simulink model "multicarFS_spacingError"  (R2019a)
settings: Solver=FixedStepAuto  StartTime=0.0  StopTime=600  FixedStep=0.01  RelTol=1e-3
libraries: simulink x14, autolibshared x8, vehdynlibsteering x8, autolibutils x8, eeGeneralControl x7
(part 1 of 2)
settings Model: Creator=ckreienk  LastModifiedBy=ckreienk

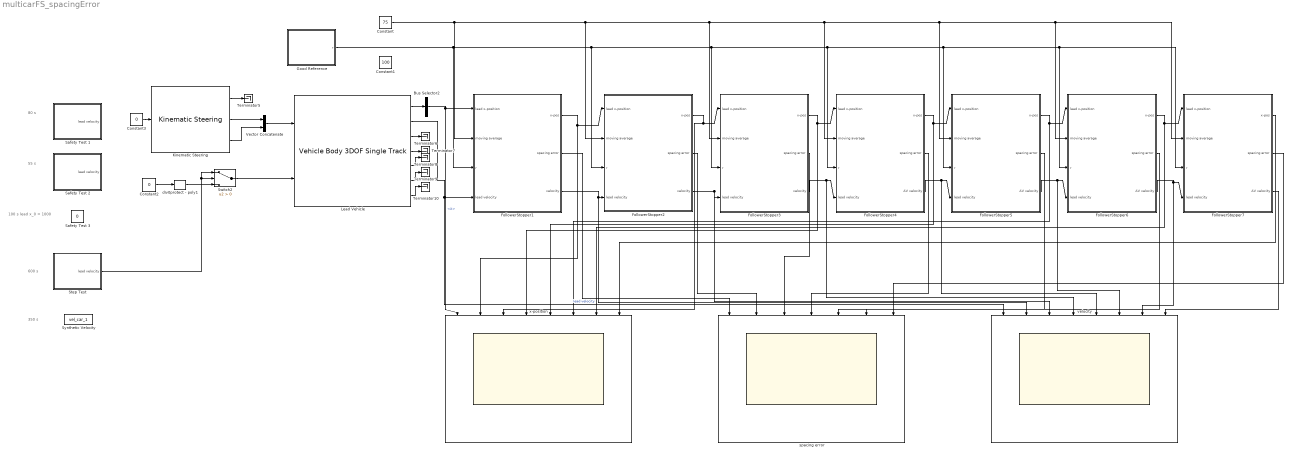
== system multicarFS_spacingError ==
  note: 600 s
  note: 100 s
      | lead x_0 = 1000
  note: 55 s
  note: 350 s
  note: 80 s
  Bus Selector2 : BusSelector  OutputSignals=InertFrm.Geom.Disp.X
  Constant : Constant  Value=75
  Constant1 : Constant  Value=100
  Constant2 : Constant  Value=0
  Constant3 : Constant  Value=0
  FollowerStopper1 : Subsystem
  FollowerStopper2 : Subsystem
  FollowerStopper3 : Subsystem
  FollowerStopper4 : Subsystem
  FollowerStopper5 : Subsystem
  FollowerStopper6 : Subsystem
  FollowerStopper7 : Subsystem
  Good Reference : Subsystem
  Kinematic Steering : vehdynlibsteering/Kinematic Steering  StrgType=Ackerman  StrgRatioType=Constant  Loc=Front  NrmlFctr=0.01  TrckWdth=1  WhlBase=1.524  Db=0  StrgRng=1.25*pi  StrgAngBpts="[-6.2832   -5.0265   -3.7699   -2.5133   -1.2566         0    1.2566    2.5133    3.7699    5.0265    6.2832]"  StrgRatioTbl=|  StrgRatio=100  StrgArmLngth=0.1  RckCsLngth=0.5  TieRodLngth=0.248  D=0.2  PnnRadius=0.0057  PnnRadiusTbl="[0.0055    0.0055    0.0056    0.0057    0.0058    0.0057    0.0057    0.0057    0.0056    0.0055    0.0055]"  RodLngth=0.1  ParaArmLngth=0.9  aMode=2
      | [13.5000   13.3750   13.2500   13.1250   13.0000   13.0000   13.0000   13.1250   13.2500   13.3750   13.5000
      | ]
      settings: SourceProductName=Vehicle Dynamics Blockset
  Lead Vehicle : autolibshared/Vehicle Body 3DOF Single Track  trackMode=Dual  inputMode=External longitudinal velocity  frontSteerMode=on  rearSteerMode=off  windMode=off  muMode=off  extFMode=off  extMMode=off  extXo=off  extpsio=off  extxdoto=off  extro=off  extYo=off  extTamb=off  extydoto=off  aMode=2  NF=2  NR=2  m=2000  a=1.4  b=1.6  h=0.35  X_o=80  xdot_o=0  CalphaMode=off  sigmaMode=on  d=0  w=[1.4,1.4]  Cy_f=12e3  Cy_r=11e3  sigma_f=.1  sigma_r=.1  alpha_f_brk=[-.1 .1]  Cy_f_data=[-9e3 9e3]  alpha_r_brk=[-.1 .1]  Cy_r_data=[-9e3 9e3]  Y_o=0  ydot_o=0  Izz=4000  psi_o=0  r_o=0  Af=2  Cd=.3  Cl=.1  Cpm=.1  beta_w=[0:0.01:0.3]  Cs=[0:0.03:0.9]  Cym=[0:0.01:0.3]  Pabs=101325  Tair=273  g=9.81  mu=1  xdot_tol=.01  Fznom=5000  Fxtire_sat=7e4  Fytire_sat=7e4  longOff=0  latOff=0  vertOff=0  wrapAng=off
      settings: SourceProductName=Powertrain Blockset  SourceProductBaseCode=PW
  Safety Test 1 : Subsystem
  Safety Test 2 : Subsystem
  Safety Test 3 : Constant  Value=0
  Step Test : Subsystem
  Switch2 : Switch  Criteria=u2 > Threshold
  Synthetic Velocity : FromWorkspace  VariableName=vel_car_1
  Terminator{5..10} (6 alike) : Terminator
  Vector Concatenate : Concatenate
  div0protect - poly1 : autolibutils/div0protect - poly  thresh=1e-3  aMode=2
      settings: SourceProductName=Powertrain Blockset  SourceProductBaseCode=PW
  spacing error : Scope  NumInputPorts=7
  velocity : Scope  NumInputPorts=8
  x-position : Scope  NumInputPorts=8
  wires:
  Constant3/1 -> Kinematic Steering/1
  Switch2/1 -> Lead Vehicle/2
  Kinematic Steering/3 -> Vector Concatenate/2
  div0protect - poly1/1 -> Switch2/3
  Lead Vehicle/6 -> Terminator9/1
  Step Test/1(lead velocity) -> Switch2/1, Switch2/2
  Kinematic Steering/2 -> Vector Concatenate/1
  Lead Vehicle/7 -> Terminator10/1
  Lead Vehicle/3 -> Terminator6/1
  Lead Vehicle/4 -> Terminator7/1
  Constant2/1 -> div0protect - poly1/1
  Kinematic Steering/1 -> Terminator5/1
  Vector Concatenate/1 -> Lead Vehicle/1
  Lead Vehicle/2 -> velocity/1, FollowerStopper1/4(lead velocity)  "lead velocity"
  Lead Vehicle/5 -> Terminator8/1
  Bus Selector2/1 -> FollowerStopper1/1(lead x-position), x-position/1  "<X>"
  Lead Vehicle/1 -> Bus Selector2/1
  FollowerStopper1/1(x-pos) -> x-position/2, FollowerStopper2/1(lead x-position)
  FollowerStopper1/3(velocity) -> velocity/2, FollowerStopper2/4(lead velocity)
  FollowerStopper2/1(x-pos) -> x-position/3, FollowerStopper3/1(lead x-position)
  FollowerStopper2/3(velocity) -> FollowerStopper3/4(lead velocity), velocity/3
  FollowerStopper3/1(x-pos) -> x-position/4, FollowerStopper4/1(lead x-position)
  FollowerStopper3/3(velocity) -> velocity/4, FollowerStopper4/4(lead velocity)
  FollowerStopper4/1(x-pos) -> x-position/5, FollowerStopper5/1(lead x-position)
  FollowerStopper4/3(AV velocity) -> velocity/5, FollowerStopper5/4(lead velocity)
  FollowerStopper5/1(x-pos) -> x-position/6, FollowerStopper6/1(lead x-position)
  FollowerStopper5/3(AV velocity) -> velocity/6, FollowerStopper6/4(lead velocity)
  FollowerStopper6/1(x-pos) -> x-position/7, FollowerStopper7/1(lead x-position)
  FollowerStopper6/3(AV velocity) -> velocity/7, FollowerStopper7/4(lead velocity)
  FollowerStopper7/1(x-pos) -> x-position/8
  FollowerStopper6/2(spacing error) -> spacing error/6
  FollowerStopper3/2(spacing error) -> spacing error/3
  FollowerStopper2/2(spacing error) -> spacing error/2
  FollowerStopper5/2(spacing error) -> spacing error/5
  FollowerStopper7/2(spacing error) -> spacing error/7
  FollowerStopper1/2(spacing error) -> spacing error/1
  FollowerStopper4/2(spacing error) -> spacing error/4
  FollowerStopper7/3(AV velocity) -> velocity/8
  Constant/1 -> FollowerStopper7/2(moving average), FollowerStopper6/2(moving average), FollowerStopper5/2(moving average), FollowerStopper4/2(moving average), FollowerStopper3/2(moving average), FollowerStopper2/2(moving average), FollowerStopper1/2(moving average)
  Good Reference/1(r) -> FollowerStopper6/3(r), FollowerStopper7/3(r), FollowerStopper5/3(r), FollowerStopper4/3(r), FollowerStopper3/3(r), FollowerStopper2/3(r), FollowerStopper1/3(r)

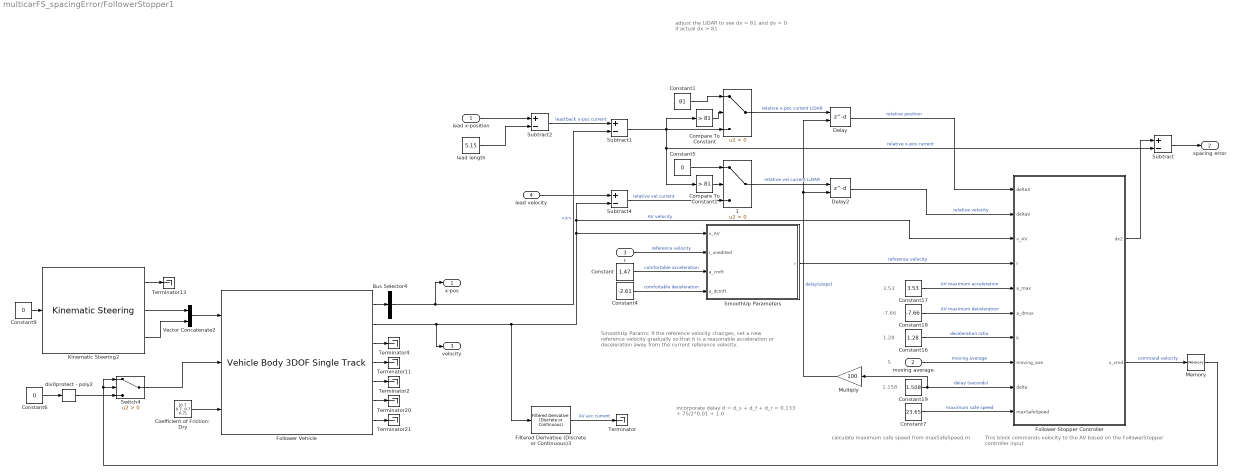
== system multicarFS_spacingError/FollowerStopper1 ==
  note: -7.66
  note: 5
  note: 1.158
  note: adjust the LiDAR to see
      | dx = 81 and dv = 0
      | if actual dx > 81
  note: incorporate delay
      | d = d_s + d_f + d_r
      | = 0.133 + 75/2*0.01 + 1.0
  note: SmoothUp Params:
      | If the reference velocity changes,
      | set a new reference velocity gradually
      | so that it is a reasonable acceleration
      | or deceleration away from the current
      | reference velocity.
  note: This block commands velocity to the AV based
      | on the FollowerStopper controller input
  note: calculate maximum safe speed
      | from maxSafeSpeed.m
  note: 3.53
  note: 1.28
  lead x-position : Inport
  moving average : Inport  Port=2
  r : Inport  Port=3
  lead velocity : Inport  Port=4
  " " : Switch  Criteria=u2 > Threshold
  " 1" : Switch  Criteria=u2 > Threshold
  Bus Selector4 : BusSelector  OutputSignals=InertFrm.Geom.Disp.X
  Coefficient of Friction: Dry : Constant  Value=[0.7 0.7; 0.7 0.7]
  Compare To Constant : simulink/Logic and Bit Operations/Compare To Constant  relop=>  const=81  OutDataTypeStr=boolean
  Compare To Constant1 : simulink/Logic and Bit Operations/Compare To Constant  relop=>  const=81  OutDataTypeStr=boolean
  Constant : Constant  Value=1.47
  Constant1 : Constant  Value=81
  Constant16 : Constant  Value=1.28
  Constant17 : Constant  Value=3.53
  Constant18 : Constant  Value=-7.66
  Constant19 : Constant  Value=1.508
  Constant4 : Constant  Value=-2.61
  Constant5 : Constant  Value=0
  Constant6 : Constant  Value=0
  Constant7 : Constant  Value=23.65
  Constant9 : Constant  Value=0
  Delay : Delay  DelayLengthSource=Input port  DelayLength=183
      settings: InputPortMap=u0,p1
  Delay2 : Delay  DelayLengthSource=Input port  DelayLength=183
      settings: InputPortMap=u0,p1
  Filtered Derivative (Discrete or Continuous)3 : eeGeneralControl/Filtered Derivative (Discrete or Continuous)  K=1  T=0.1  B=20  A=-20  minRatio=10  Ts=-1
      settings: SourceProductName=Simscape Electrical  SourceProductBaseCode=PS
  Follower Stopper Controller : Subsystem
  Follower Vehicle : autolibshared/Vehicle Body 3DOF Single Track  trackMode=Dual  inputMode=External longitudinal velocity  frontSteerMode=on  rearSteerMode=off  windMode=off  muMode=on  extFMode=off  extMMode=off  extXo=off  extpsio=off  extxdoto=off  extro=off  extYo=off  extTamb=off  extydoto=off  aMode=2  NF=2  NR=2  m=2000  a=1.4  b=1.6  h=0.35  X_o=70  xdot_o=0  CalphaMode=off  sigmaMode=on  d=0  w=[1.4,1.4]  Cy_f=12e3  Cy_r=11e3  sigma_f=.1  sigma_r=.1  alpha_f_brk=[-.1 .1]  Cy_f_data=[-9e3 9e3]  alpha_r_brk=[-.1 .1]  Cy_r_data=[-9e3 9e3]  Y_o=0  ydot_o=0  Izz=4000  psi_o=0  r_o=0  Af=2  Cd=.3  Cl=.1  Cpm=.1  beta_w=[0:0.01:0.3]  Cs=[0:0.03:0.9]  Cym=[0:0.01:0.3]  Pabs=101325  Tair=273  g=9.81  mu=1  xdot_tol=.01  Fznom=5000  Fxtire_sat=7e4  Fytire_sat=7e4  longOff=0  latOff=0  vertOff=0  wrapAng=off
      settings: SourceProductName=Powertrain Blockset  SourceProductBaseCode=PW
  Kinematic Steering2 : vehdynlibsteering/Kinematic Steering  StrgType=Ackerman  StrgRatioType=Constant  Loc=Front  NrmlFctr=0.01  TrckWdth=1  WhlBase=1.524  Db=0  StrgRng=1.25*pi  StrgAngBpts="[-6.2832   -5.0265   -3.7699   -2.5133   -1.2566         0    1.2566    2.5133    3.7699    5.0265    6.2832]"  StrgRatioTbl=|  StrgRatio=100  StrgArmLngth=0.1  RckCsLngth=0.5  TieRodLngth=0.248  D=0.2  PnnRadius=0.0057  PnnRadiusTbl="[0.0055    0.0055    0.0056    0.0057    0.0058    0.0057    0.0057    0.0057    0.0056    0.0055    0.0055]"  RodLngth=0.1  ParaArmLngth=0.9  aMode=2
      | [13.5000   13.3750   13.2500   13.1250   13.0000   13.0000   13.0000   13.1250   13.2500   13.3750   13.5000
      | ]
      settings: SourceProductName=Vehicle Dynamics Blockset
  Memory : Memory
  Multiply : Gain  Gain=100
  SmoothUp Parameters : MATLAB Function  TreatAsAtomicUnit=on
  Subtract{,1..2,4} (4 alike) : Sum  Inputs=+-
  Switch4 : Switch  Criteria=u2 > Threshold
  Terminator{,2,4,11,13,20..21} (7 alike) : Terminator
  Vector Concatenate2 : Concatenate
  div0protect - poly2 : autolibutils/div0protect - poly  thresh=1e-3  aMode=2
      settings: SourceProductName=Powertrain Blockset  SourceProductBaseCode=PW
  lead length : Constant  Value=5.15
  x-pos : Outport
  spacing error : Outport  Port=2
  velocity : Outport  Port=3
  wires:
  Vector Concatenate2/1 -> Follower Vehicle/1
  Bus Selector4/1 -> x-pos/1, Subtract1/2  "<X>"
  Subtract2/1 -> Subtract1/1  "lead back x-pos current"
  div0protect - poly2/1 -> Switch4/3
  Constant7/1 -> Follower Stopper Controller/10(maxSafeSpeed)  "maximum safe speed"
  Follower Vehicle/3 -> Terminator4/1
  Kinematic Steering2/2 -> Vector Concatenate2/1
  Subtract4/1 -> " 1"/3  "relative vel current"
  lead x-position/1 -> Subtract2/1
  Constant6/1 -> div0protect - poly2/1
  Switch4/1 -> Follower Vehicle/2
  Kinematic Steering2/3 -> Vector Concatenate2/2
  Constant4/1 -> SmoothUp Parameters/4(a_dcmft)  "comfortable deceleration"
  Follower Vehicle/2 -> velocity/1, Filtered Derivative (Discrete or Continuous)3/1, SmoothUp Parameters/1(v_AV), Follower Stopper Controller/3(v_AV), Subtract4/2  "AV velocity"
  Constant19/1 -> Multiply/1, Follower Stopper Controller/9(delta)  "delay (seconds)"
  Constant9/1 -> Kinematic Steering2/1
  Constant5/1 -> " 1"/1
  Constant1/1 -> " "/1
  Subtract1/1 -> Compare To Constant1/1, Subtract/2, Compare To Constant/1, " "/3  "relative x-pos current"
  Follower Vehicle/1 -> Bus Selector4/1
  Memory/1 -> Switch4/1, Switch4/2
  Follower Vehicle/4 -> Terminator11/1
  " 1"/1 -> Delay2/1  "relative vel current LiDAR"
  Delay/1 -> Follower Stopper Controller/1(deltaX)  "relative position"
  SmoothUp Parameters/1(r) -> Follower Stopper Controller/4(r)  "reference velocity"
  Delay2/1 -> Follower Stopper Controller/2(deltaV)  "relative velocity"
  Multiply/1 -> Delay2/2, Delay/2  "delay(steps)"
  Follower Vehicle/5 -> Terminator2/1
  Constant17/1 -> Follower Stopper Controller/5(a_max)  "AV maximum acceleration"
  lead length/1 -> Subtract2/2
  Constant16/1 -> Follower Stopper Controller/7(k)  "deceleration ratio"
  moving average/1 -> Follower Stopper Controller/8(moving_ave)  "moving average"
  lead velocity/1 -> Subtract4/1
  Kinematic Steering2/1 -> Terminator13/1
  Follower Vehicle/6 -> Terminator20/1
  Follower Stopper Controller/2(v_cmd) -> Memory/1  "command velocity"
  Coefficient of Friction: Dry/1 -> Follower Vehicle/3
  Compare To Constant/1 -> " "/2
  Constant18/1 -> Follower Stopper Controller/6(a_dmax)  "AV maximum deceleration"
  Constant/1 -> SmoothUp Parameters/3(a_cmft)  "comfortable acceleration"
  " "/1 -> Delay/1  "relative x-pos current LiDAR"
  r/1 -> SmoothUp Parameters/2(r_unedited)  "reference velocity"
  Compare To Constant1/1 -> " 1"/2
  Follower Vehicle/7 -> Terminator21/1
  Filtered Derivative (Discrete or Continuous)3/1 -> Terminator/1  "AV acc current"
  Follower Stopper Controller/1(dx2) -> Subtract/1
  Subtract/1 -> spacing error/1

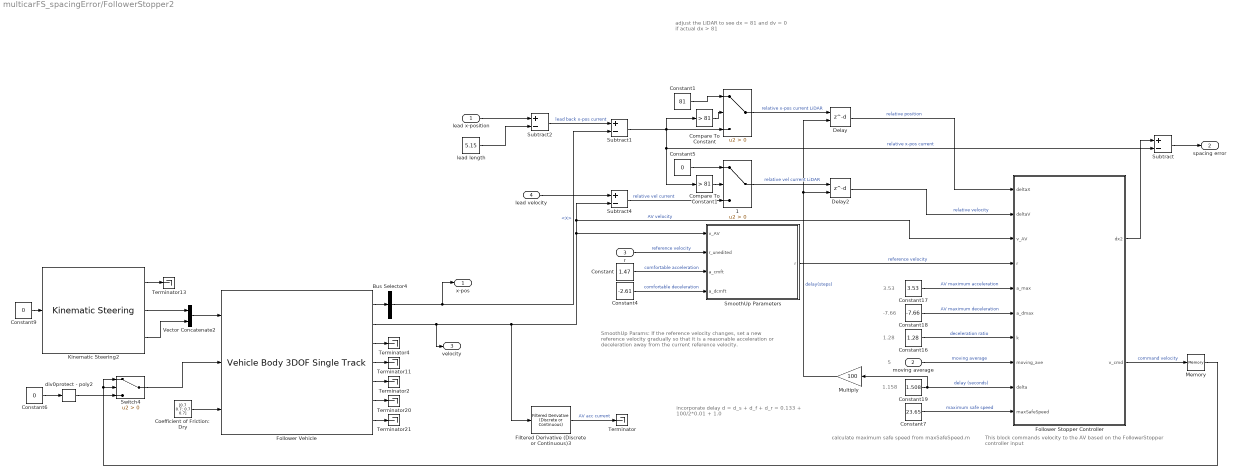
== system multicarFS_spacingError/FollowerStopper2 ==
  note: 1.28
  note: 3.53
  note: calculate maximum safe speed
      | from maxSafeSpeed.m
  note: This block commands velocity to the AV based
      | on the FollowerStopper controller input
  note: SmoothUp Params:
      | If the reference velocity changes,
      | set a new reference velocity gradually
      | so that it is a reasonable acceleration
      | or deceleration away from the current
      | reference velocity.
  note: incorporate delay
      | d = d_s + d_f + d_r
      | = 0.133 + 100/2*0.01 + 1.0
  note: adjust the LiDAR to see
      | dx = 81 and dv = 0
      | if actual dx > 81
  note: 1.158
  note: 5
  note: -7.66
  lead x-position : Inport
  moving average : Inport  Port=2
  r : Inport  Port=3
  lead velocity : Inport  Port=4
  " " : Switch  Criteria=u2 > Threshold
  " 1" : Switch  Criteria=u2 > Threshold
  Bus Selector4 : BusSelector  OutputSignals=InertFrm.Geom.Disp.X
  Coefficient of Friction: Dry : Constant  Value=[0.7 0.7; 0.7 0.7]
  Compare To Constant : simulink/Logic and Bit Operations/Compare To Constant  relop=>  const=81  OutDataTypeStr=boolean
  Compare To Constant1 : simulink/Logic and Bit Operations/Compare To Constant  relop=>  const=81  OutDataTypeStr=boolean
  Constant : Constant  Value=1.47
  Constant1 : Constant  Value=81
  Constant16 : Constant  Value=1.28
  Constant17 : Constant  Value=3.53
  Constant18 : Constant  Value=-7.66
  Constant19 : Constant  Value=1.508
  Constant4 : Constant  Value=-2.61
  Constant5 : Constant  Value=0
  Constant6 : Constant  Value=0
  Constant7 : Constant  Value=23.65
  Constant9 : Constant  Value=0
  Delay : Delay  DelayLengthSource=Input port  DelayLength=183
      settings: InputPortMap=u0,p1
  Delay2 : Delay  DelayLengthSource=Input port  DelayLength=183
      settings: InputPortMap=u0,p1
  Filtered Derivative (Discrete or Continuous)3 : eeGeneralControl/Filtered Derivative (Discrete or Continuous)  K=1  T=0.1  B=20  A=-20  minRatio=10  Ts=-1
      settings: SourceProductName=Simscape Electrical  SourceProductBaseCode=PS
  Follower Stopper Controller : Subsystem
  Follower Vehicle : autolibshared/Vehicle Body 3DOF Single Track  trackMode=Dual  inputMode=External longitudinal velocity  frontSteerMode=on  rearSteerMode=off  windMode=off  muMode=on  extFMode=off  extMMode=off  extXo=off  extpsio=off  extxdoto=off  extro=off  extYo=off  extTamb=off  extydoto=off  aMode=2  NF=2  NR=2  m=2000  a=1.4  b=1.6  h=0.35  X_o=60  xdot_o=0  CalphaMode=off  sigmaMode=on  d=0  w=[1.4,1.4]  Cy_f=12e3  Cy_r=11e3  sigma_f=.1  sigma_r=.1  alpha_f_brk=[-.1 .1]  Cy_f_data=[-9e3 9e3]  alpha_r_brk=[-.1 .1]  Cy_r_data=[-9e3 9e3]  Y_o=0  ydot_o=0  Izz=4000  psi_o=0  r_o=0  Af=2  Cd=.3  Cl=.1  Cpm=.1  beta_w=[0:0.01:0.3]  Cs=[0:0.03:0.9]  Cym=[0:0.01:0.3]  Pabs=101325  Tair=273  g=9.81  mu=1  xdot_tol=.01  Fznom=5000  Fxtire_sat=7e4  Fytire_sat=7e4  longOff=0  latOff=0  vertOff=0  wrapAng=off
      settings: SourceProductName=Powertrain Blockset  SourceProductBaseCode=PW
  Kinematic Steering2 : vehdynlibsteering/Kinematic Steering  StrgType=Ackerman  StrgRatioType=Constant  Loc=Front  NrmlFctr=0.01  TrckWdth=1  WhlBase=1.524  Db=0  StrgRng=1.25*pi  StrgAngBpts="[-6.2832   -5.0265   -3.7699   -2.5133   -1.2566         0    1.2566    2.5133    3.7699    5.0265    6.2832]"  StrgRatioTbl=|  StrgRatio=100  StrgArmLngth=0.1  RckCsLngth=0.5  TieRodLngth=0.248  D=0.2  PnnRadius=0.0057  PnnRadiusTbl="[0.0055    0.0055    0.0056    0.0057    0.0058    0.0057    0.0057    0.0057    0.0056    0.0055    0.0055]"  RodLngth=0.1  ParaArmLngth=0.9  aMode=2
      | [13.5000   13.3750   13.2500   13.1250   13.0000   13.0000   13.0000   13.1250   13.2500   13.3750   13.5000
      | ]
      settings: SourceProductName=Vehicle Dynamics Blockset
  Memory : Memory
  Multiply : Gain  Gain=100
  SmoothUp Parameters : MATLAB Function  TreatAsAtomicUnit=on
  Subtract{,1..2,4} (4 alike) : Sum  Inputs=+-
  Switch4 : Switch  Criteria=u2 > Threshold
  Terminator{,2,4,11,13,20..21} (7 alike) : Terminator
  Vector Concatenate2 : Concatenate
  div0protect - poly2 : autolibutils/div0protect - poly  thresh=1e-3  aMode=2
      settings: SourceProductName=Powertrain Blockset  SourceProductBaseCode=PW
  lead length : Constant  Value=5.15
  x-pos : Outport
  spacing error : Outport  Port=2
  velocity : Outport  Port=3
  wires:
  Subtract/1 -> spacing error/1
  Follower Stopper Controller/1(dx2) -> Subtract/1
  Filtered Derivative (Discrete or Continuous)3/1 -> Terminator/1  "AV acc current"
  Follower Vehicle/7 -> Terminator21/1
  Compare To Constant1/1 -> " 1"/2
  r/1 -> SmoothUp Parameters/2(r_unedited)  "reference velocity"
  " "/1 -> Delay/1  "relative x-pos current LiDAR"
  Constant/1 -> SmoothUp Parameters/3(a_cmft)  "comfortable acceleration"
  Constant18/1 -> Follower Stopper Controller/6(a_dmax)  "AV maximum deceleration"
  Compare To Constant/1 -> " "/2
  Coefficient of Friction: Dry/1 -> Follower Vehicle/3
  Follower Stopper Controller/2(v_cmd) -> Memory/1  "command velocity"
  Follower Vehicle/6 -> Terminator20/1
  Kinematic Steering2/1 -> Terminator13/1
  lead velocity/1 -> Subtract4/1
  moving average/1 -> Follower Stopper Controller/8(moving_ave)  "moving average"
  Constant16/1 -> Follower Stopper Controller/7(k)  "deceleration ratio"
  lead length/1 -> Subtract2/2
  Constant17/1 -> Follower Stopper Controller/5(a_max)  "AV maximum acceleration"
  Follower Vehicle/5 -> Terminator2/1
  Multiply/1 -> Delay/2, Delay2/2  "delay(steps)"
  Delay2/1 -> Follower Stopper Controller/2(deltaV)  "relative velocity"
  SmoothUp Parameters/1(r) -> Follower Stopper Controller/4(r)  "reference velocity"
  Delay/1 -> Follower Stopper Controller/1(deltaX)  "relative position"
  " 1"/1 -> Delay2/1  "relative vel current LiDAR"
  Follower Vehicle/4 -> Terminator11/1
  Memory/1 -> Switch4/2, Switch4/1
  Follower Vehicle/1 -> Bus Selector4/1
  Subtract1/1 -> " "/3, Compare To Constant/1, Subtract/2, Compare To Constant1/1  "relative x-pos current"
  Constant1/1 -> " "/1
  Constant5/1 -> " 1"/1
  Constant9/1 -> Kinematic Steering2/1
  Constant19/1 -> Follower Stopper Controller/9(delta), Multiply/1  "delay (seconds)"
  Follower Vehicle/2 -> Subtract4/2, Follower Stopper Controller/3(v_AV), SmoothUp Parameters/1(v_AV), Filtered Derivative (Discrete or Continuous)3/1, velocity/1  "AV velocity"
  Constant4/1 -> SmoothUp Parameters/4(a_dcmft)  "comfortable deceleration"
  Kinematic Steering2/3 -> Vector Concatenate2/2
  Switch4/1 -> Follower Vehicle/2
  Constant6/1 -> div0protect - poly2/1
  lead x-position/1 -> Subtract2/1
  Subtract4/1 -> " 1"/3  "relative vel current"
  Kinematic Steering2/2 -> Vector Concatenate2/1
  Follower Vehicle/3 -> Terminator4/1
  Constant7/1 -> Follower Stopper Controller/10(maxSafeSpeed)  "maximum safe speed"
  div0protect - poly2/1 -> Switch4/3
  Subtract2/1 -> Subtract1/1  "lead back x-pos current"
  Bus Selector4/1 -> x-pos/1, Subtract1/2  "<X>"
  Vector Concatenate2/1 -> Follower Vehicle/1

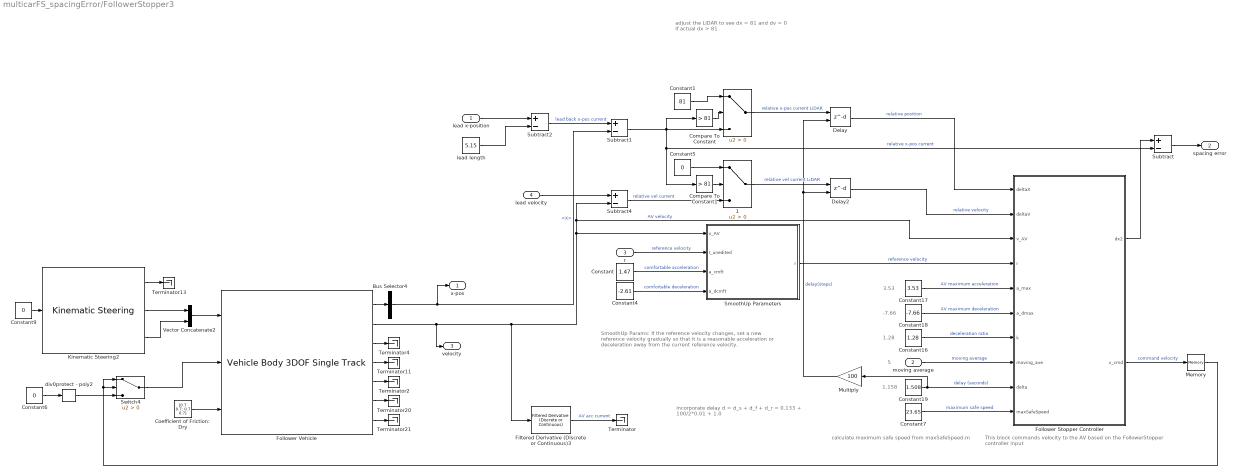
== system multicarFS_spacingError/FollowerStopper3 ==
  note: -7.66
  note: 5
  note: 1.158
  note: adjust the LiDAR to see
      | dx = 81 and dv = 0
      | if actual dx > 81
  note: incorporate delay
      | d = d_s + d_f + d_r
      | = 0.133 + 100/2*0.01 + 1.0
  note: SmoothUp Params:
      | If the reference velocity changes,
      | set a new reference velocity gradually
      | so that it is a reasonable acceleration
      | or deceleration away from the current
      | reference velocity.
  note: This block commands velocity to the AV based
      | on the FollowerStopper controller input
  note: calculate maximum safe speed
      | from maxSafeSpeed.m
  note: 3.53
  note: 1.28
  lead x-position : Inport
  moving average : Inport  Port=2
  r : Inport  Port=3
  lead velocity : Inport  Port=4
  " " : Switch  Criteria=u2 > Threshold
  " 1" : Switch  Criteria=u2 > Threshold
  Bus Selector4 : BusSelector  OutputSignals=InertFrm.Geom.Disp.X
  Coefficient of Friction: Dry : Constant  Value=[0.7 0.7; 0.7 0.7]
  Compare To Constant : simulink/Logic and Bit Operations/Compare To Constant  relop=>  const=81  OutDataTypeStr=boolean
  Compare To Constant1 : simulink/Logic and Bit Operations/Compare To Constant  relop=>  const=81  OutDataTypeStr=boolean
  Constant : Constant  Value=1.47
  Constant1 : Constant  Value=81
  Constant16 : Constant  Value=1.28
  Constant17 : Constant  Value=3.53
  Constant18 : Constant  Value=-7.66
  Constant19 : Constant  Value=1.508
  Constant4 : Constant  Value=-2.61
  Constant5 : Constant  Value=0
  Constant6 : Constant  Value=0
  Constant7 : Constant  Value=23.65
  Constant9 : Constant  Value=0
  Delay : Delay  DelayLengthSource=Input port  DelayLength=183
      settings: InputPortMap=u0,p1
  Delay2 : Delay  DelayLengthSource=Input port  DelayLength=183
      settings: InputPortMap=u0,p1
  Filtered Derivative (Discrete or Continuous)3 : eeGeneralControl/Filtered Derivative (Discrete or Continuous)  K=1  T=0.1  B=20  A=-20  minRatio=10  Ts=-1
      settings: SourceProductName=Simscape Electrical  SourceProductBaseCode=PS
  Follower Stopper Controller : Subsystem
  Follower Vehicle : autolibshared/Vehicle Body 3DOF Single Track  trackMode=Dual  inputMode=External longitudinal velocity  frontSteerMode=on  rearSteerMode=off  windMode=off  muMode=on  extFMode=off  extMMode=off  extXo=off  extpsio=off  extxdoto=off  extro=off  extYo=off  extTamb=off  extydoto=off  aMode=2  NF=2  NR=2  m=2000  a=1.4  b=1.6  h=0.35  X_o=50  xdot_o=0  CalphaMode=off  sigmaMode=on  d=0  w=[1.4,1.4]  Cy_f=12e3  Cy_r=11e3  sigma_f=.1  sigma_r=.1  alpha_f_brk=[-.1 .1]  Cy_f_data=[-9e3 9e3]  alpha_r_brk=[-.1 .1]  Cy_r_data=[-9e3 9e3]  Y_o=0  ydot_o=0  Izz=4000  psi_o=0  r_o=0  Af=2  Cd=.3  Cl=.1  Cpm=.1  beta_w=[0:0.01:0.3]  Cs=[0:0.03:0.9]  Cym=[0:0.01:0.3]  Pabs=101325  Tair=273  g=9.81  mu=1  xdot_tol=.01  Fznom=5000  Fxtire_sat=7e4  Fytire_sat=7e4  longOff=0  latOff=0  vertOff=0  wrapAng=off
      settings: SourceProductName=Powertrain Blockset  SourceProductBaseCode=PW
  Kinematic Steering2 : vehdynlibsteering/Kinematic Steering  StrgType=Ackerman  StrgRatioType=Constant  Loc=Front  NrmlFctr=0.01  TrckWdth=1  WhlBase=1.524  Db=0  StrgRng=1.25*pi  StrgAngBpts="[-6.2832   -5.0265   -3.7699   -2.5133   -1.2566         0    1.2566    2.5133    3.7699    5.0265    6.2832]"  StrgRatioTbl=|  StrgRatio=100  StrgArmLngth=0.1  RckCsLngth=0.5  TieRodLngth=0.248  D=0.2  PnnRadius=0.0057  PnnRadiusTbl="[0.0055    0.0055    0.0056    0.0057    0.0058    0.0057    0.0057    0.0057    0.0056    0.0055    0.0055]"  RodLngth=0.1  ParaArmLngth=0.9  aMode=2
      | [13.5000   13.3750   13.2500   13.1250   13.0000   13.0000   13.0000   13.1250   13.2500   13.3750   13.5000
      | ]
      settings: SourceProductName=Vehicle Dynamics Blockset
  Memory : Memory
  Multiply : Gain  Gain=100
  SmoothUp Parameters : MATLAB Function  TreatAsAtomicUnit=on
  Subtract{,1..2,4} (4 alike) : Sum  Inputs=+-
  Switch4 : Switch  Criteria=u2 > Threshold
  Terminator{,2,4,11,13,20..21} (7 alike) : Terminator
  Vector Concatenate2 : Concatenate
  div0protect - poly2 : autolibutils/div0protect - poly  thresh=1e-3  aMode=2
      settings: SourceProductName=Powertrain Blockset  SourceProductBaseCode=PW
  lead length : Constant  Value=5.15
  x-pos : Outport
  spacing error : Outport  Port=2
  velocity : Outport  Port=3
  wires:
  Vector Concatenate2/1 -> Follower Vehicle/1
  Bus Selector4/1 -> x-pos/1, Subtract1/2  "<X>"
  Subtract2/1 -> Subtract1/1  "lead back x-pos current"
  div0protect - poly2/1 -> Switch4/3
  Constant7/1 -> Follower Stopper Controller/10(maxSafeSpeed)  "maximum safe speed"
  Follower Vehicle/3 -> Terminator4/1
  Kinematic Steering2/2 -> Vector Concatenate2/1
  Subtract4/1 -> " 1"/3  "relative vel current"
  lead x-position/1 -> Subtract2/1
  Constant6/1 -> div0protect - poly2/1
  Switch4/1 -> Follower Vehicle/2
  Kinematic Steering2/3 -> Vector Concatenate2/2
  Constant4/1 -> SmoothUp Parameters/4(a_dcmft)  "comfortable deceleration"
  Follower Vehicle/2 -> velocity/1, Filtered Derivative (Discrete or Continuous)3/1, SmoothUp Parameters/1(v_AV), Follower Stopper Controller/3(v_AV), Subtract4/2  "AV velocity"
  Constant19/1 -> Multiply/1, Follower Stopper Controller/9(delta)  "delay (seconds)"
  Constant9/1 -> Kinematic Steering2/1
  Constant5/1 -> " 1"/1
  Constant1/1 -> " "/1
  Subtract1/1 -> Compare To Constant1/1, Subtract/2, Compare To Constant/1, " "/3  "relative x-pos current"
  Follower Vehicle/1 -> Bus Selector4/1
  Memory/1 -> Switch4/1, Switch4/2
  Follower Vehicle/4 -> Terminator11/1
  " 1"/1 -> Delay2/1  "relative vel current LiDAR"
  Delay/1 -> Follower Stopper Controller/1(deltaX)  "relative position"
  SmoothUp Parameters/1(r) -> Follower Stopper Controller/4(r)  "reference velocity"
  Delay2/1 -> Follower Stopper Controller/2(deltaV)  "relative velocity"
  Multiply/1 -> Delay2/2, Delay/2  "delay(steps)"
  Follower Vehicle/5 -> Terminator2/1
  Constant17/1 -> Follower Stopper Controller/5(a_max)  "AV maximum acceleration"
  lead length/1 -> Subtract2/2
  Constant16/1 -> Follower Stopper Controller/7(k)  "deceleration ratio"
  moving average/1 -> Follower Stopper Controller/8(moving_ave)  "moving average"
  lead velocity/1 -> Subtract4/1
  Kinematic Steering2/1 -> Terminator13/1
  Follower Vehicle/6 -> Terminator20/1
  Follower Stopper Controller/2(v_cmd) -> Memory/1  "command velocity"
  Coefficient of Friction: Dry/1 -> Follower Vehicle/3
  Compare To Constant/1 -> " "/2
  Constant18/1 -> Follower Stopper Controller/6(a_dmax)  "AV maximum deceleration"
  Constant/1 -> SmoothUp Parameters/3(a_cmft)  "comfortable acceleration"
  " "/1 -> Delay/1  "relative x-pos current LiDAR"
  r/1 -> SmoothUp Parameters/2(r_unedited)  "reference velocity"
  Compare To Constant1/1 -> " 1"/2
  Follower Vehicle/7 -> Terminator21/1
  Filtered Derivative (Discrete or Continuous)3/1 -> Terminator/1  "AV acc current"
  Follower Stopper Controller/1(dx2) -> Subtract/1
  Subtract/1 -> spacing error/1

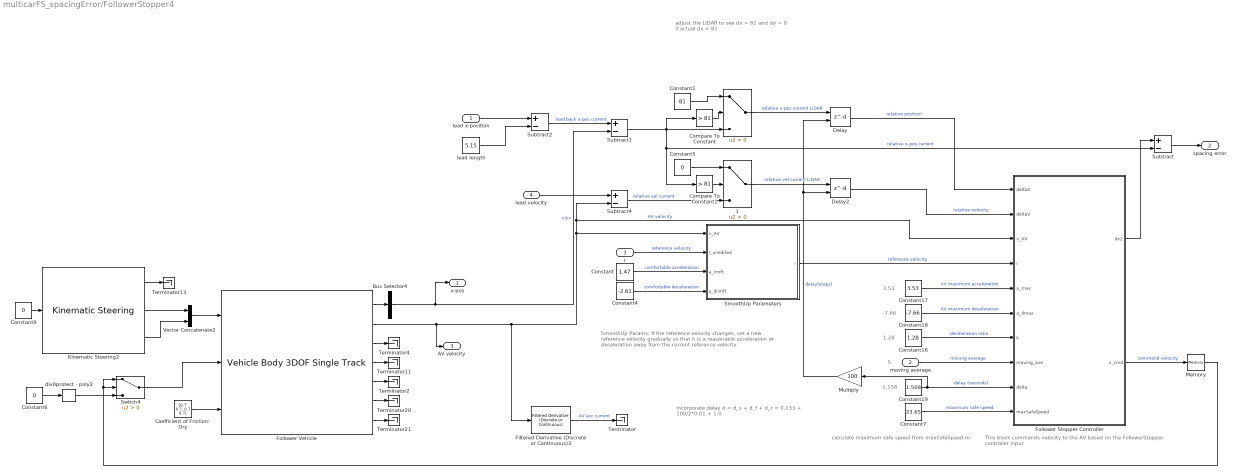
== system multicarFS_spacingError/FollowerStopper4 ==
  note: 1.28
  note: 3.53
  note: calculate maximum safe speed
      | from maxSafeSpeed.m
  note: This block commands velocity to the AV based
      | on the FollowerStopper controller input
  note: SmoothUp Params:
      | If the reference velocity changes,
      | set a new reference velocity gradually
      | so that it is a reasonable acceleration
      | or deceleration away from the current
      | reference velocity.
  note: incorporate delay
      | d = d_s + d_f + d_r
      | = 0.133 + 100/2*0.01 + 1.0
  note: adjust the LiDAR to see
      | dx = 81 and dv = 0
      | if actual dx > 81
  note: 1.158
  note: 5
  note: -7.66
  lead x-position : Inport
  moving average : Inport  Port=2
  r : Inport  Port=3
  lead velocity : Inport  Port=4
  " " : Switch  Criteria=u2 > Threshold
  " 1" : Switch  Criteria=u2 > Threshold
  Bus Selector4 : BusSelector  OutputSignals=InertFrm.Geom.Disp.X
  Coefficient of Friction: Dry : Constant  Value=[0.7 0.7; 0.7 0.7]
  Compare To Constant : simulink/Logic and Bit Operations/Compare To Constant  relop=>  const=81  OutDataTypeStr=boolean
  Compare To Constant1 : simulink/Logic and Bit Operations/Compare To Constant  relop=>  const=81  OutDataTypeStr=boolean
  Constant : Constant  Value=1.47
  Constant1 : Constant  Value=81
  Constant16 : Constant  Value=1.28
  Constant17 : Constant  Value=3.53
  Constant18 : Constant  Value=-7.66
  Constant19 : Constant  Value=1.508
  Constant4 : Constant  Value=-2.61
  Constant5 : Constant  Value=0
  Constant6 : Constant  Value=0
  Constant7 : Constant  Value=23.65
  Constant9 : Constant  Value=0
  Delay : Delay  DelayLengthSource=Input port  DelayLength=183
      settings: InputPortMap=u0,p1
  Delay2 : Delay  DelayLengthSource=Input port  DelayLength=183
      settings: InputPortMap=u0,p1
  Filtered Derivative (Discrete or Continuous)3 : eeGeneralControl/Filtered Derivative (Discrete or Continuous)  K=1  T=0.1  B=20  A=-20  minRatio=10  Ts=-1
      settings: SourceProductName=Simscape Electrical  SourceProductBaseCode=PS
  Follower Stopper Controller : Subsystem
  Follower Vehicle : autolibshared/Vehicle Body 3DOF Single Track  trackMode=Dual  inputMode=External longitudinal velocity  frontSteerMode=on  rearSteerMode=off  windMode=off  muMode=on  extFMode=off  extMMode=off  extXo=off  extpsio=off  extxdoto=off  extro=off  extYo=off  extTamb=off  extydoto=off  aMode=2  NF=2  NR=2  m=2000  a=1.4  b=1.6  h=0.35  X_o=40  xdot_o=0  CalphaMode=off  sigmaMode=on  d=0  w=[1.4,1.4]  Cy_f=12e3  Cy_r=11e3  sigma_f=.1  sigma_r=.1  alpha_f_brk=[-.1 .1]  Cy_f_data=[-9e3 9e3]  alpha_r_brk=[-.1 .1]  Cy_r_data=[-9e3 9e3]  Y_o=0  ydot_o=0  Izz=4000  psi_o=0  r_o=0  Af=2  Cd=.3  Cl=.1  Cpm=.1  beta_w=[0:0.01:0.3]  Cs=[0:0.03:0.9]  Cym=[0:0.01:0.3]  Pabs=101325  Tair=273  g=9.81  mu=1  xdot_tol=.01  Fznom=5000  Fxtire_sat=7e4  Fytire_sat=7e4  longOff=0  latOff=0  vertOff=0  wrapAng=off
      settings: SourceProductName=Powertrain Blockset  SourceProductBaseCode=PW
  Kinematic Steering2 : vehdynlibsteering/Kinematic Steering  StrgType=Ackerman  StrgRatioType=Constant  Loc=Front  NrmlFctr=0.01  TrckWdth=1  WhlBase=1.524  Db=0  StrgRng=1.25*pi  StrgAngBpts="[-6.2832   -5.0265   -3.7699   -2.5133   -1.2566         0    1.2566    2.5133    3.7699    5.0265    6.2832]"  StrgRatioTbl=|  StrgRatio=100  StrgArmLngth=0.1  RckCsLngth=0.5  TieRodLngth=0.248  D=0.2  PnnRadius=0.0057  PnnRadiusTbl="[0.0055    0.0055    0.0056    0.0057    0.0058    0.0057    0.0057    0.0057    0.0056    0.0055    0.0055]"  RodLngth=0.1  ParaArmLngth=0.9  aMode=2
      | [13.5000   13.3750   13.2500   13.1250   13.0000   13.0000   13.0000   13.1250   13.2500   13.3750   13.5000
      | ]
      settings: SourceProductName=Vehicle Dynamics Blockset
  Memory : Memory
  Multiply : Gain  Gain=100
  SmoothUp Parameters : MATLAB Function  TreatAsAtomicUnit=on
  Subtract{,1..2,4} (4 alike) : Sum  Inputs=+-
  Switch4 : Switch  Criteria=u2 > Threshold
  Terminator{,2,4,11,13,20..21} (7 alike) : Terminator
  Vector Concatenate2 : Concatenate
  div0protect - poly2 : autolibutils/div0protect - poly  thresh=1e-3  aMode=2
      settings: SourceProductName=Powertrain Blockset  SourceProductBaseCode=PW
  lead length : Constant  Value=5.15
  x-pos : Outport
  spacing error : Outport  Port=2
  AV velocity : Outport  Port=3
  wires:
  Subtract/1 -> spacing error/1
  Follower Stopper Controller/1(dx2) -> Subtract/1
  Filtered Derivative (Discrete or Continuous)3/1 -> Terminator/1  "AV acc current"
  Follower Vehicle/7 -> Terminator21/1
  Compare To Constant1/1 -> " 1"/2
  r/1 -> SmoothUp Parameters/2(r_unedited)  "reference velocity"
  " "/1 -> Delay/1  "relative x-pos current LiDAR"
  Constant/1 -> SmoothUp Parameters/3(a_cmft)  "comfortable acceleration"
  Constant18/1 -> Follower Stopper Controller/6(a_dmax)  "AV maximum deceleration"
  Compare To Constant/1 -> " "/2
  Coefficient of Friction: Dry/1 -> Follower Vehicle/3
  Follower Stopper Controller/2(v_cmd) -> Memory/1  "command velocity"
  Follower Vehicle/6 -> Terminator20/1
  Kinematic Steering2/1 -> Terminator13/1
  lead velocity/1 -> Subtract4/1
  moving average/1 -> Follower Stopper Controller/8(moving_ave)  "moving average"
  Constant16/1 -> Follower Stopper Controller/7(k)  "deceleration ratio"
  lead length/1 -> Subtract2/2
  Constant17/1 -> Follower Stopper Controller/5(a_max)  "AV maximum acceleration"
  Follower Vehicle/5 -> Terminator2/1
  Multiply/1 -> Delay/2, Delay2/2  "delay(steps)"
  Delay2/1 -> Follower Stopper Controller/2(deltaV)  "relative velocity"
  SmoothUp Parameters/1(r) -> Follower Stopper Controller/4(r)  "reference velocity"
  Delay/1 -> Follower Stopper Controller/1(deltaX)  "relative position"
  " 1"/1 -> Delay2/1  "relative vel current LiDAR"
  Follower Vehicle/4 -> Terminator11/1
  Memory/1 -> Switch4/2, Switch4/1
  Follower Vehicle/1 -> Bus Selector4/1
  Subtract1/1 -> " "/3, Compare To Constant/1, Subtract/2, Compare To Constant1/1  "relative x-pos current"
  Constant1/1 -> " "/1
  Constant5/1 -> " 1"/1
  Constant9/1 -> Kinematic Steering2/1
  Constant19/1 -> Follower Stopper Controller/9(delta), Multiply/1  "delay (seconds)"
  Follower Vehicle/2 -> Subtract4/2, Follower Stopper Controller/3(v_AV), SmoothUp Parameters/1(v_AV), Filtered Derivative (Discrete or Continuous)3/1, AV velocity/1  "AV velocity"
  Constant4/1 -> SmoothUp Parameters/4(a_dcmft)  "comfortable deceleration"
  Kinematic Steering2/3 -> Vector Concatenate2/2
  Switch4/1 -> Follower Vehicle/2
  Constant6/1 -> div0protect - poly2/1
  lead x-position/1 -> Subtract2/1
  Subtract4/1 -> " 1"/3  "relative vel current"
  Kinematic Steering2/2 -> Vector Concatenate2/1
  Follower Vehicle/3 -> Terminator4/1
  Constant7/1 -> Follower Stopper Controller/10(maxSafeSpeed)  "maximum safe speed"
  div0protect - poly2/1 -> Switch4/3
  Subtract2/1 -> Subtract1/1  "lead back x-pos current"
  Bus Selector4/1 -> x-pos/1, Subtract1/2  "<X>"
  Vector Concatenate2/1 -> Follower Vehicle/1

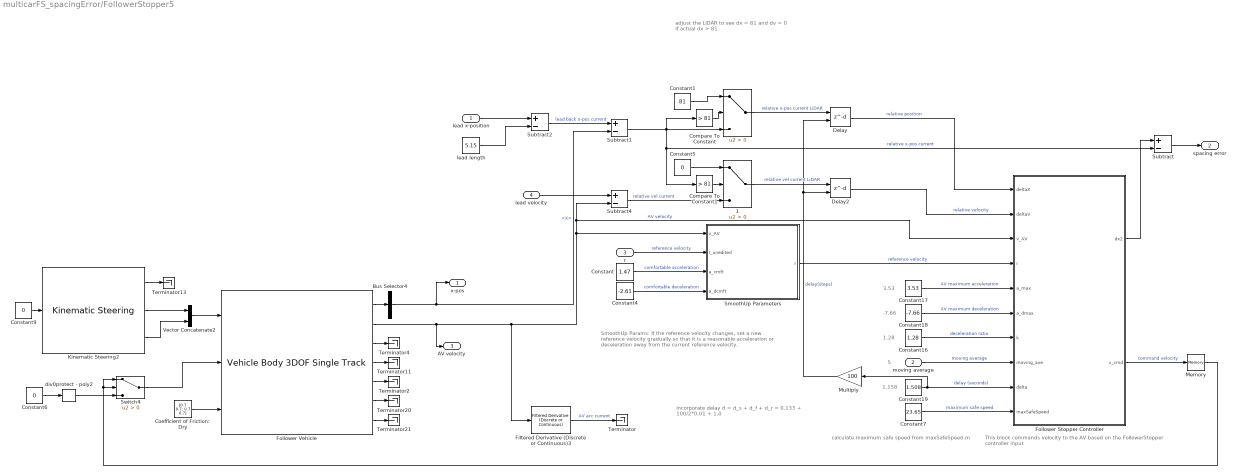
== system multicarFS_spacingError/FollowerStopper5 ==
  note: -7.66
  note: 5
  note: 1.158
  note: adjust the LiDAR to see
      | dx = 81 and dv = 0
      | if actual dx > 81
  note: incorporate delay
      | d = d_s + d_f + d_r
      | = 0.133 + 100/2*0.01 + 1.0
  note: SmoothUp Params:
      | If the reference velocity changes,
      | set a new reference velocity gradually
      | so that it is a reasonable acceleration
      | or deceleration away from the current
      | reference velocity.
  note: This block commands velocity to the AV based
      | on the FollowerStopper controller input
  note: calculate maximum safe speed
      | from maxSafeSpeed.m
  note: 3.53
  note: 1.28
  lead x-position : Inport
  moving average : Inport  Port=2
  r : Inport  Port=3
  lead velocity : Inport  Port=4
  " " : Switch  Criteria=u2 > Threshold
  " 1" : Switch  Criteria=u2 > Threshold
  Bus Selector4 : BusSelector  OutputSignals=InertFrm.Geom.Disp.X
  Coefficient of Friction: Dry : Constant  Value=[0.7 0.7; 0.7 0.7]
  Compare To Constant : simulink/Logic and Bit Operations/Compare To Constant  relop=>  const=81  OutDataTypeStr=boolean
  Compare To Constant1 : simulink/Logic and Bit Operations/Compare To Constant  relop=>  const=81  OutDataTypeStr=boolean
  Constant : Constant  Value=1.47
  Constant1 : Constant  Value=81
  Constant16 : Constant  Value=1.28
  Constant17 : Constant  Value=3.53
  Constant18 : Constant  Value=-7.66
  Constant19 : Constant  Value=1.508
  Constant4 : Constant  Value=-2.61
  Constant5 : Constant  Value=0
  Constant6 : Constant  Value=0
  Constant7 : Constant  Value=23.65
  Constant9 : Constant  Value=0
  Delay : Delay  DelayLengthSource=Input port  DelayLength=183
      settings: InputPortMap=u0,p1
  Delay2 : Delay  DelayLengthSource=Input port  DelayLength=183
      settings: InputPortMap=u0,p1
  Filtered Derivative (Discrete or Continuous)3 : eeGeneralControl/Filtered Derivative (Discrete or Continuous)  K=1  T=0.1  B=20  A=-20  minRatio=10  Ts=-1
      settings: SourceProductName=Simscape Electrical  SourceProductBaseCode=PS
  Follower Stopper Controller : Subsystem
  Follower Vehicle : autolibshared/Vehicle Body 3DOF Single Track  trackMode=Dual  inputMode=External longitudinal velocity  frontSteerMode=on  rearSteerMode=off  windMode=off  muMode=on  extFMode=off  extMMode=off  extXo=off  extpsio=off  extxdoto=off  extro=off  extYo=off  extTamb=off  extydoto=off  aMode=2  NF=2  NR=2  m=2000  a=1.4  b=1.6  h=0.35  X_o=30  xdot_o=0  CalphaMode=off  sigmaMode=on  d=0  w=[1.4,1.4]  Cy_f=12e3  Cy_r=11e3  sigma_f=.1  sigma_r=.1  alpha_f_brk=[-.1 .1]  Cy_f_data=[-9e3 9e3]  alpha_r_brk=[-.1 .1]  Cy_r_data=[-9e3 9e3]  Y_o=0  ydot_o=0  Izz=4000  psi_o=0  r_o=0  Af=2  Cd=.3  Cl=.1  Cpm=.1  beta_w=[0:0.01:0.3]  Cs=[0:0.03:0.9]  Cym=[0:0.01:0.3]  Pabs=101325  Tair=273  g=9.81  mu=1  xdot_tol=.01  Fznom=5000  Fxtire_sat=7e4  Fytire_sat=7e4  longOff=0  latOff=0  vertOff=0  wrapAng=off
      settings: SourceProductName=Powertrain Blockset  SourceProductBaseCode=PW
  Kinematic Steering2 : vehdynlibsteering/Kinematic Steering  StrgType=Ackerman  StrgRatioType=Constant  Loc=Front  NrmlFctr=0.01  TrckWdth=1  WhlBase=1.524  Db=0  StrgRng=1.25*pi  StrgAngBpts="[-6.2832   -5.0265   -3.7699   -2.5133   -1.2566         0    1.2566    2.5133    3.7699    5.0265    6.2832]"  StrgRatioTbl=|  StrgRatio=100  StrgArmLngth=0.1  RckCsLngth=0.5  TieRodLngth=0.248  D=0.2  PnnRadius=0.0057  PnnRadiusTbl="[0.0055    0.0055    0.0056    0.0057    0.0058    0.0057    0.0057    0.0057    0.0056    0.0055    0.0055]"  RodLngth=0.1  ParaArmLngth=0.9  aMode=2
      | [13.5000   13.3750   13.2500   13.1250   13.0000   13.0000   13.0000   13.1250   13.2500   13.3750   13.5000
      | ]
      settings: SourceProductName=Vehicle Dynamics Blockset
  Memory : Memory
  Multiply : Gain  Gain=100
  SmoothUp Parameters : MATLAB Function  TreatAsAtomicUnit=on
  Subtract{,1..2,4} (4 alike) : Sum  Inputs=+-
  Switch4 : Switch  Criteria=u2 > Threshold
  Terminator{,2,4,11,13,20..21} (7 alike) : Terminator
  Vector Concatenate2 : Concatenate
  div0protect - poly2 : autolibutils/div0protect - poly  thresh=1e-3  aMode=2
      settings: SourceProductName=Powertrain Blockset  SourceProductBaseCode=PW
  lead length : Constant  Value=5.15
  x-pos : Outport
  spacing error : Outport  Port=2
  AV velocity : Outport  Port=3
  wires:
  Vector Concatenate2/1 -> Follower Vehicle/1
  Bus Selector4/1 -> x-pos/1, Subtract1/2  "<X>"
  Subtract2/1 -> Subtract1/1  "lead back x-pos current"
  div0protect - poly2/1 -> Switch4/3
  Constant7/1 -> Follower Stopper Controller/10(maxSafeSpeed)  "maximum safe speed"
  Follower Vehicle/3 -> Terminator4/1
  Kinematic Steering2/2 -> Vector Concatenate2/1
  Subtract4/1 -> " 1"/3  "relative vel current"
  lead x-position/1 -> Subtract2/1
  Constant6/1 -> div0protect - poly2/1
  Switch4/1 -> Follower Vehicle/2
  Kinematic Steering2/3 -> Vector Concatenate2/2
  Constant4/1 -> SmoothUp Parameters/4(a_dcmft)  "comfortable deceleration"
  Follower Vehicle/2 -> AV velocity/1, Filtered Derivative (Discrete or Continuous)3/1, SmoothUp Parameters/1(v_AV), Follower Stopper Controller/3(v_AV), Subtract4/2  "AV velocity"
  Constant19/1 -> Multiply/1, Follower Stopper Controller/9(delta)  "delay (seconds)"
  Constant9/1 -> Kinematic Steering2/1
  Constant5/1 -> " 1"/1
  Constant1/1 -> " "/1
  Subtract1/1 -> Compare To Constant1/1, Subtract/2, Compare To Constant/1, " "/3  "relative x-pos current"
  Follower Vehicle/1 -> Bus Selector4/1
  Memory/1 -> Switch4/1, Switch4/2
  Follower Vehicle/4 -> Terminator11/1
  " 1"/1 -> Delay2/1  "relative vel current LiDAR"
  Delay/1 -> Follower Stopper Controller/1(deltaX)  "relative position"
  SmoothUp Parameters/1(r) -> Follower Stopper Controller/4(r)  "reference velocity"
  Delay2/1 -> Follower Stopper Controller/2(deltaV)  "relative velocity"
  Multiply/1 -> Delay2/2, Delay/2  "delay(steps)"
  Follower Vehicle/5 -> Terminator2/1
  Constant17/1 -> Follower Stopper Controller/5(a_max)  "AV maximum acceleration"
  lead length/1 -> Subtract2/2
  Constant16/1 -> Follower Stopper Controller/7(k)  "deceleration ratio"
  moving average/1 -> Follower Stopper Controller/8(moving_ave)  "moving average"
  lead velocity/1 -> Subtract4/1
  Kinematic Steering2/1 -> Terminator13/1
  Follower Vehicle/6 -> Terminator20/1
  Follower Stopper Controller/2(v_cmd) -> Memory/1  "command velocity"
  Coefficient of Friction: Dry/1 -> Follower Vehicle/3
  Compare To Constant/1 -> " "/2
  Constant18/1 -> Follower Stopper Controller/6(a_dmax)  "AV maximum deceleration"
  Constant/1 -> SmoothUp Parameters/3(a_cmft)  "comfortable acceleration"
  " "/1 -> Delay/1  "relative x-pos current LiDAR"
  r/1 -> SmoothUp Parameters/2(r_unedited)  "reference velocity"
  Compare To Constant1/1 -> " 1"/2
  Follower Vehicle/7 -> Terminator21/1
  Filtered Derivative (Discrete or Continuous)3/1 -> Terminator/1  "AV acc current"
  Follower Stopper Controller/1(dx2) -> Subtract/1
  Subtract/1 -> spacing error/1

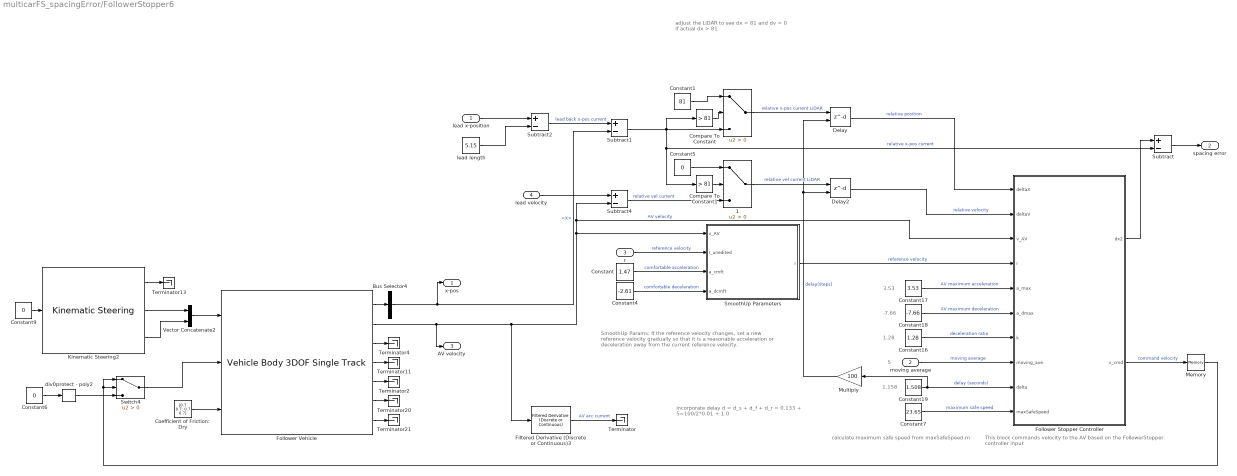
== system multicarFS_spacingError/FollowerStopper6 ==
  note: 1.28
  note: 3.53
  note: calculate maximum safe speed
      | from maxSafeSpeed.m
  note: This block commands velocity to the AV based
      | on the FollowerStopper controller input
  note: SmoothUp Params:
      | If the reference velocity changes,
      | set a new reference velocity gradually
      | so that it is a reasonable acceleration
      | or deceleration away from the current
      | reference velocity.
  note: incorporate delay
      | d = d_s + d_f + d_r
      | = 0.133 + 5=100/2*0.01 + 1.0
  note: adjust the LiDAR to see
      | dx = 81 and dv = 0
      | if actual dx > 81
  note: 1.158
  note: 5
  note: -7.66
  lead x-position : Inport
  moving average : Inport  Port=2
  r : Inport  Port=3
  lead velocity : Inport  Port=4
  " " : Switch  Criteria=u2 > Threshold
  " 1" : Switch  Criteria=u2 > Threshold
  Bus Selector4 : BusSelector  OutputSignals=InertFrm.Geom.Disp.X
  Coefficient of Friction: Dry : Constant  Value=[0.7 0.7; 0.7 0.7]
  Compare To Constant : simulink/Logic and Bit Operations/Compare To Constant  relop=>  const=81  OutDataTypeStr=boolean
  Compare To Constant1 : simulink/Logic and Bit Operations/Compare To Constant  relop=>  const=81  OutDataTypeStr=boolean
  Constant : Constant  Value=1.47
  Constant1 : Constant  Value=81
  Constant16 : Constant  Value=1.28
  Constant17 : Constant  Value=3.53
  Constant18 : Constant  Value=-7.66
  Constant19 : Constant  Value=1.508
  Constant4 : Constant  Value=-2.61
  Constant5 : Constant  Value=0
  Constant6 : Constant  Value=0
  Constant7 : Constant  Value=23.65
  Constant9 : Constant  Value=0
  Delay : Delay  DelayLengthSource=Input port  DelayLength=183
      settings: InputPortMap=u0,p1
  Delay2 : Delay  DelayLengthSource=Input port  DelayLength=183
      settings: InputPortMap=u0,p1
  Filtered Derivative (Discrete or Continuous)3 : eeGeneralControl/Filtered Derivative (Discrete or Continuous)  K=1  T=0.1  B=20  A=-20  minRatio=10  Ts=-1
      settings: SourceProductName=Simscape Electrical  SourceProductBaseCode=PS
  Follower Stopper Controller : Subsystem
  Follower Vehicle : autolibshared/Vehicle Body 3DOF Single Track  trackMode=Dual  inputMode=External longitudinal velocity  frontSteerMode=on  rearSteerMode=off  windMode=off  muMode=on  extFMode=off  extMMode=off  extXo=off  extpsio=off  extxdoto=off  extro=off  extYo=off  extTamb=off  extydoto=off  aMode=2  NF=2  NR=2  m=2000  a=1.4  b=1.6  h=0.35  X_o=20  xdot_o=0  CalphaMode=off  sigmaMode=on  d=0  w=[1.4,1.4]  Cy_f=12e3  Cy_r=11e3  sigma_f=.1  sigma_r=.1  alpha_f_brk=[-.1 .1]  Cy_f_data=[-9e3 9e3]  alpha_r_brk=[-.1 .1]  Cy_r_data=[-9e3 9e3]  Y_o=0  ydot_o=0  Izz=4000  psi_o=0  r_o=0  Af=2  Cd=.3  Cl=.1  Cpm=.1  beta_w=[0:0.01:0.3]  Cs=[0:0.03:0.9]  Cym=[0:0.01:0.3]  Pabs=101325  Tair=273  g=9.81  mu=1  xdot_tol=.01  Fznom=5000  Fxtire_sat=7e4  Fytire_sat=7e4  longOff=0  latOff=0  vertOff=0  wrapAng=off
      settings: SourceProductName=Powertrain Blockset  SourceProductBaseCode=PW
  Kinematic Steering2 : vehdynlibsteering/Kinematic Steering  StrgType=Ackerman  StrgRatioType=Constant  Loc=Front  NrmlFctr=0.01  TrckWdth=1  WhlBase=1.524  Db=0  StrgRng=1.25*pi  StrgAngBpts="[-6.2832   -5.0265   -3.7699   -2.5133   -1.2566         0    1.2566    2.5133    3.7699    5.0265    6.2832]"  StrgRatioTbl=|  StrgRatio=100  StrgArmLngth=0.1  RckCsLngth=0.5  TieRodLngth=0.248  D=0.2  PnnRadius=0.0057  PnnRadiusTbl="[0.0055    0.0055    0.0056    0.0057    0.0058    0.0057    0.0057    0.0057    0.0056    0.0055    0.0055]"  RodLngth=0.1  ParaArmLngth=0.9  aMode=2
      | [13.5000   13.3750   13.2500   13.1250   13.0000   13.0000   13.0000   13.1250   13.2500   13.3750   13.5000
      | ]
      settings: SourceProductName=Vehicle Dynamics Blockset
  Memory : Memory
  Multiply : Gain  Gain=100
  SmoothUp Parameters : MATLAB Function  TreatAsAtomicUnit=on
  Subtract{,1..2,4} (4 alike) : Sum  Inputs=+-
  Switch4 : Switch  Criteria=u2 > Threshold
  Terminator{,2,4,11,13,20..21} (7 alike) : Terminator
  Vector Concatenate2 : Concatenate
  div0protect - poly2 : autolibutils/div0protect - poly  thresh=1e-3  aMode=2
      settings: SourceProductName=Powertrain Blockset  SourceProductBaseCode=PW
  lead length : Constant  Value=5.15
  x-pos : Outport
  spacing error : Outport  Port=2
  AV velocity : Outport  Port=3
  wires:
  Subtract/1 -> spacing error/1
  Follower Stopper Controller/1(dx2) -> Subtract/1
  Filtered Derivative (Discrete or Continuous)3/1 -> Terminator/1  "AV acc current"
  Follower Vehicle/7 -> Terminator21/1
  Compare To Constant1/1 -> " 1"/2
  r/1 -> SmoothUp Parameters/2(r_unedited)  "reference velocity"
  " "/1 -> Delay/1  "relative x-pos current LiDAR"
  Constant/1 -> SmoothUp Parameters/3(a_cmft)  "comfortable acceleration"
  Constant18/1 -> Follower Stopper Controller/6(a_dmax)  "AV maximum deceleration"
  Compare To Constant/1 -> " "/2
  Coefficient of Friction: Dry/1 -> Follower Vehicle/3
  Follower Stopper Controller/2(v_cmd) -> Memory/1  "command velocity"
  Follower Vehicle/6 -> Terminator20/1
  Kinematic Steering2/1 -> Terminator13/1
  lead velocity/1 -> Subtract4/1
  moving average/1 -> Follower Stopper Controller/8(moving_ave)  "moving average"
  Constant16/1 -> Follower Stopper Controller/7(k)  "deceleration ratio"
  lead length/1 -> Subtract2/2
  Constant17/1 -> Follower Stopper Controller/5(a_max)  "AV maximum acceleration"
  Follower Vehicle/5 -> Terminator2/1
  Multiply/1 -> Delay/2, Delay2/2  "delay(steps)"
  Delay2/1 -> Follower Stopper Controller/2(deltaV)  "relative velocity"
  SmoothUp Parameters/1(r) -> Follower Stopper Controller/4(r)  "reference velocity"
  Delay/1 -> Follower Stopper Controller/1(deltaX)  "relative position"
  " 1"/1 -> Delay2/1  "relative vel current LiDAR"
  Follower Vehicle/4 -> Terminator11/1
  Memory/1 -> Switch4/2, Switch4/1
  Follower Vehicle/1 -> Bus Selector4/1
  Subtract1/1 -> " "/3, Compare To Constant/1, Subtract/2, Compare To Constant1/1  "relative x-pos current"
  Constant1/1 -> " "/1
  Constant5/1 -> " 1"/1
  Constant9/1 -> Kinematic Steering2/1
  Constant19/1 -> Follower Stopper Controller/9(delta), Multiply/1  "delay (seconds)"
  Follower Vehicle/2 -> Subtract4/2, Follower Stopper Controller/3(v_AV), SmoothUp Parameters/1(v_AV), Filtered Derivative (Discrete or Continuous)3/1, AV velocity/1  "AV velocity"
  Constant4/1 -> SmoothUp Parameters/4(a_dcmft)  "comfortable deceleration"
  Kinematic Steering2/3 -> Vector Concatenate2/2
  Switch4/1 -> Follower Vehicle/2
  Constant6/1 -> div0protect - poly2/1
  lead x-position/1 -> Subtract2/1
  Subtract4/1 -> " 1"/3  "relative vel current"
  Kinematic Steering2/2 -> Vector Concatenate2/1
  Follower Vehicle/3 -> Terminator4/1
  Constant7/1 -> Follower Stopper Controller/10(maxSafeSpeed)  "maximum safe speed"
  div0protect - poly2/1 -> Switch4/3
  Subtract2/1 -> Subtract1/1  "lead back x-pos current"
  Bus Selector4/1 -> x-pos/1, Subtract1/2  "<X>"
  Vector Concatenate2/1 -> Follower Vehicle/1
